simulink model "CFGOC_SSPUT02"  (R2023b)
settings: Solver=FixedStepAuto  StartTime=0.0  StopTime=400  RelTol=1e-3  EnableMultiTasking=on
undefined symbols (not defined in the file): Ta_p, Ta_x, Ta_y
libraries: mbedblockslib x11, simulink x10, mssSimulink x4, simulink_extras x2
settings Model: ExtModeTrigDuration=10  Creator=The MathWorks, Inc.  LastModifiedBy=Ly Soi
settings SolverCC: AlgebraicLoopSolver=TrustRegion  AutoInsertRateTranBlk=on  MaxZcPerStep=1
settings DataIOCC: ReturnWorkspaceOutputs=off
settings OptimizationCC: MaxStackSize=64
settings DebuggingCC: MultiTaskRateTransMsg=warning  ParameterTunabilityLossMsg=error  UnconnectedInputMsg=warning  UnconnectedOutputMsg=warning  UnconnectedLineMsg=warning  SubsystemReferenceDiagnosticForUnitTest=warning  ArithmeticOperatorsInVariantConditions=warning
settings HardwareCC: ProdBitPerPointer=32  ProdBitPerSizeT=32  ProdBitPerPtrDiffT=32  ProdLargestAtomicInteger=Long  ProdLargestAtomicFloat=Double  ProdWordSize=32  ProdLongLongMode=on  ProdHWDeviceType=ARM Compatible->ARM Cortex
settings ModelReferenceCC: EnableRefExpFcnMdlSchedulingChecks=on
settings SFSimCC: SimUseLocalCustomCode=off
settings RTWCC: Description=Embedded Coder  SystemTargetFile=ert.tlc  HardwareBoard=STM32 Nucleo F746ZG  TemplateMakefile=ert_default_tmf  GenerateReport=on  RTWUseLocalCustomCode=off  Toolchain=GNU Tools for ARM Embedded Processors  LaunchReport=on  DLArmComputeVersion=19.05
settings CodeAppCC: ForceParamTrailComments=on  OperatorAnnotations=on  StateflowObjectComments=on  MATLABSourceComments=on
settings ERTTargetCC: CodeReplacementLibrary=ARM Cortex-M (Optimized)  MultiwordLength=2048  ERTCustomFileBanners=off  SupportContinuousTime=on  SupportNonInlinedSFcns=on  RemoveResetFunc=off  ModelStepFunctionPrototypeControlCompliant=off  ExtModeTransport=3  ExtModeStaticAlloc=on  ExtModeStaticAllocSize=2000  ExtModeMexFile=ext_xcp  ExtModeIntrfLevel=Level2 - Open  ERTSrcFileBannerTemplate=codertarget_code_template.cgt  ERTHdrFileBannerTemplate=codertarget_code_template.cgt  ERTDataSrcFileTemplate=codertarget_code_template.cgt  ERTDataHdrFileTemplate=codertarget_code_template.cgt
settings ConfigComp: CovMetricSettings=dsw  CovSaveCumulativeToWorkspaceVar=on  CovSaveSingleToWorkspaceVar=on  CovExternalEMLEnable=off

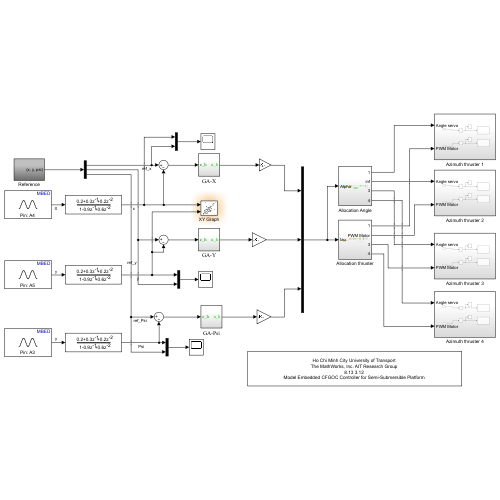
[thumbnail: Simulink's stored preview of the top-level diagram]
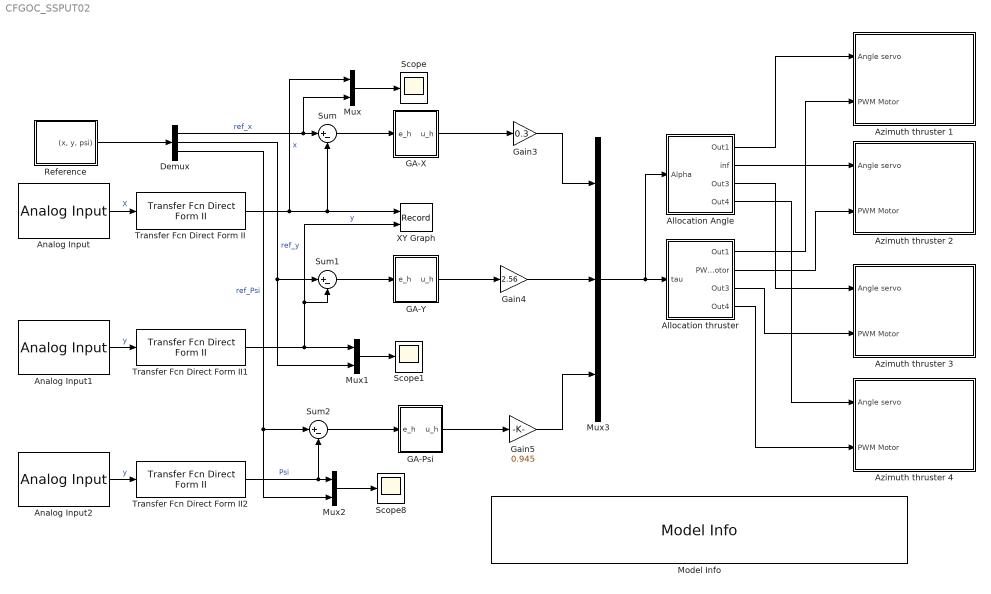
== system CFGOC_SSPUT02 ==
  Allocation Angle : Subsystem
  Allocation thruster : Subsystem
  Analog Input : mbedblockslib/Analog Input  Pin=A4  ReadResultsOnly=off  ConversionTriggerSource=Software  ExternalTriggerType=uint32( 0 )  OutputDataType=double  EnableConversionCompleteNotify=off  EnableOuputStatus=off  SampleTime=-1
      settings: LibrarySourceBlock=stmnucleorootlib/Common/Analog Input
  Analog Input1 : mbedblockslib/Analog Input  Pin=A5  ReadResultsOnly=off  ConversionTriggerSource=Software  ExternalTriggerType=uint32( 0 )  OutputDataType=double  EnableConversionCompleteNotify=off  EnableOuputStatus=off  SampleTime=-1
      settings: LibrarySourceBlock=stmnucleorootlib/Common/Analog Input
  Analog Input2 : mbedblockslib/Analog Input  Pin=A3  ReadResultsOnly=off  ConversionTriggerSource=Software  ExternalTriggerType=uint32( 0 )  OutputDataType=double  EnableConversionCompleteNotify=off  EnableOuputStatus=off  SampleTime=-1
      settings: LibrarySourceBlock=stmnucleorootlib/Common/Analog Input
  Azimuth thruster 1 : Subsystem
  Azimuth thruster 2 : Subsystem
  Azimuth thruster 3 : Subsystem
  Azimuth thruster 4 : Subsystem
  Demux : Demux  Outputs=3
  GA-Psi : Subsystem
  GA-X : Subsystem
  GA-Y : Subsystem
  Gain3 : Gain  Gain=0.3
  Gain4 : Gain  Gain=2.56
  Gain5 : Gain  Gain=0.945
  Model Info : simulink/Model-Wide Utilities/Model Info  Frame=on  DisplayStringWithTags=|  HorizontalTextAlignment=Center  LeftAlignmentValue=0.5
      | Ho Chi Minh City University of Transport
      | %<Creator> AIT Research Group
      | %<ModelVersion> 3.12
      | Model Embedded CFGOC Controller for Semi-Submersible Platform
  Mux : Mux  Inputs=2
  Mux1 : Mux  Inputs=2
  Mux2 : Mux  Inputs=2
  Mux3 : Mux  Inputs=3
  Reference : Subsystem
  Scope : Scope
  Scope1 : Scope
  Scope8 : Scope
  Sum : Sum  Inputs=|+-
  Sum1 : Sum  Inputs=|+-
  Sum2 : Sum  Inputs=|+-
  Transfer Fcn Direct Form II : simulink/Additional Math & Discrete/Additional Discrete/Transfer Fcn Direct Form II  NumCoefVec=[0.2 0.3 0.2]  DenCoefVec="[-0.9    0.6]"  vinit=0.0  DoSatur=off
  Transfer Fcn Direct Form II1 : simulink/Additional Math & Discrete/Additional Discrete/Transfer Fcn Direct Form II  NumCoefVec=[0.2 0.3 0.2]  DenCoefVec="[-0.9    0.6]"  vinit=0.0  DoSatur=off
  Transfer Fcn Direct Form II2 : simulink/Additional Math & Discrete/Additional Discrete/Transfer Fcn Direct Form II  NumCoefVec=[0.2 0.3 0.2]  DenCoefVec="[-0.9    0.6]"  vinit=0.0  DoSatur=off
  XY Graph : Record  FileSettingsInternal="{\"entries\":[{\"content\":{\"excelSettings\":{\"content\":{},\"type\":\"Streamout.ExcelSettings\"}},\"type\":\"Streamout.FileSettingStorage\",\"uuid\":\"\"}],\"packageUris\":[\"http:\\/\\/schema.mathworks.com\\/mf0\\/streamout_blocks\\/R2020a\"],\"version\":\"1.0\"}"  Layout=[1 1]  SignalsInternal="{\"entries\":[{\"content\":{\"signals\":[{\"content\":{\"blockPath\":[],\"dimensions\":[1],\"domain\":\"\",\"lineColor\":\"#a2142f\",\"plots\":[1],\"port\":1,\"signalID\":71,\"signalName\":\"Gain2\"},\"type\":\"RecordBlkView.Signal\",\"uuid\":\"\"},{\"content\":{\"blockPath\":[],\"dimensions\":[1],\"domain\":\"\",\"lineColor\":\"#139fff\",\"plots\":[1],\"port\":2,\"signalID\":74,\"signalName\":\"y\"},\"type\":\"RecordBlkView.Signal\",\"uuid\":\"\"}]},\"type\":\"RecordBlkView.InputSignals\",\"uuid\":\"\"}],\"packageUris\":[\"http:\\/\\/schema.mathworks.com\\/mf0\\/streamout_blocks\\/R2020a\"],\"version\":\"1.0\"}"  VisualizationBindings="{\"xyplotplugin\":{\"info\":[{\"series\":[{\"bindingParametersList\":[{\"parameter\":\"X-Axis\",\"signalID\":71,\"signalName\":\"Gain2\"},{\"parameter\":\"Y-Axis\",\"signalID\":74,\"signalName\":\"y\"}],\"seriesID\":16081}],\"subplotID\":1}]}}"  CompatibilityTag=XY
  wires:
  Analog Input/1 -> Transfer Fcn Direct Form II/1  "X"
  Analog Input1/1 -> Transfer Fcn Direct Form II1/1  "y"
  Demux/1 -> Mux/2, Sum/1  "ref_x"
  Demux/2 -> Mux1/2, Sum1/1  "ref_y"
  Mux/1 -> Scope/1
  Mux1/1 -> Scope1/1
  Transfer Fcn Direct Form II/1 -> Sum/2, XY Graph/1, Mux/1  "x"
  Transfer Fcn Direct Form II1/1 -> Mux1/1, XY Graph/2, Sum1/2  "y"
  GA-Psi/1(u_h) -> Gain5/1
  Sum/1 -> GA-X/1(e_h)
  Gain5/1 -> Mux3/3
  GA-Y/1(u_h) -> Gain4/1
  GA-X/1(u_h) -> Gain3/1
  Sum1/1 -> GA-Y/1(e_h)
  Gain3/1 -> Mux3/1
  Gain4/1 -> Mux3/2
  Transfer Fcn Direct Form II2/1 -> Sum2/2, Mux2/1  "Psi"
  Mux2/1 -> Scope8/1
  Analog Input2/1 -> Transfer Fcn Direct Form II2/1  "y"
  Demux/3 -> Sum2/1, Mux2/2  "ref_Psi"
  Sum2/1 -> GA-Psi/1(e_h)
  Mux3/1 -> Allocation Angle/1(Alpha), Allocation thruster/1(tau)
  Allocation Angle/1(Out1) -> Azimuth thruster 1/1(Angle servo)
  Allocation thruster/1(Out1) -> Azimuth thruster 1/2(PWM Motor)
  Allocation Angle/2(inf) -> Azimuth thruster 2/1(Angle servo)
  Allocation thruster/2(PWM Motor) -> Azimuth thruster 2/2(PWM Motor)
  Allocation Angle/3(Out3) -> Azimuth thruster 3/1(Angle servo)
  Allocation thruster/3(Out3) -> Azimuth thruster 3/2(PWM Motor)
  Allocation Angle/4(Out4) -> Azimuth thruster 4/1(Angle servo)
  Allocation thruster/4(Out4) -> Azimuth thruster 4/2(PWM Motor)
  Reference/1("(x, y, psi)") -> Demux/1

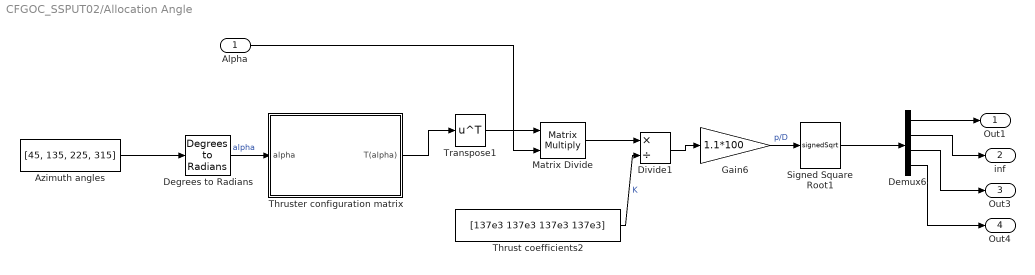
== system CFGOC_SSPUT02/Allocation Angle ==
  Alpha : Inport
  Azimuth angles : Constant  Value=[45, 135, 225, 315]
  Degrees to Radians : simulink_extras/Transformations/Degrees to Radians
  Demux6 : Demux
      settings: DisplayOption=none
  Divide1 : Product  Inputs=*/
  Gain6 : Gain  Gain=1.1*100  SaturateOnIntegerOverflow=on  OutDataTypeStr=Inherit: Same as input  ParamDataTypeStr=Inherit: Same as input
  Matrix Divide : Product  Inputs=**  Multiplication=Matrix(*)
  Signed Square Root1 : Sqrt  Operator=signedSqrt
  Thrust coefficients2 : Constant  Value=[137e3 137e3 137e3 137e3]
  "Thruster configuration matrix  " : Subsystem  AncestorBlock=mssSimulink/Modelling/Propulsion/Actuator Configuration/Thruster configuration matrix
  Transpose1 : Math  Operator=transpose
  Out1 : Outport
  inf : Outport  Port=2
  Out3 : Outport  Port=3
  Out4 : Outport  Port=4
  wires:
  Matrix Divide/1 -> Divide1/1
  Degrees to Radians/1 -> "Thruster configuration matrix  "/1(alpha)  "alpha"
  Signed Square Root1/1 -> Demux6/1
  Gain6/1 -> Signed Square Root1/1  "p/D"
  Azimuth angles/1 -> Degrees to Radians/1
  Thrust coefficients2/1 -> Divide1/2  "K"
  Transpose1/1 -> Matrix Divide/1
  Demux6/4 -> Out4/1
  Divide1/1 -> Gain6/1
  "Thruster configuration matrix  "/1(T(alpha)) -> Transpose1/1
  Alpha/1 -> Matrix Divide/2
  Demux6/1 -> Out1/1
  Demux6/3 -> Out3/1
  Demux6/2 -> inf/1

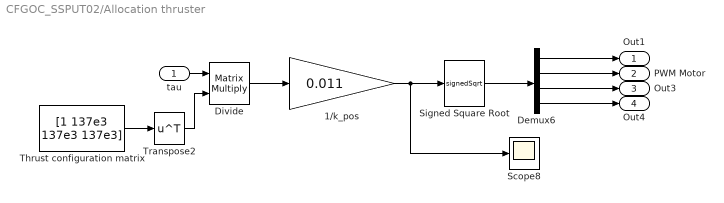
== system CFGOC_SSPUT02/Allocation thruster ==
  tau : Inport
  1/k_pos : Gain  Gain=0.011
  Demux6 : Demux
      settings: DisplayOption=none
  Divide : Product  Inputs=**  Multiplication=Matrix(*)
  Scope8 : Scope
  Signed Square Root : Sqrt  Operator=signedSqrt
  Thrust configuration matrix : Constant  Value=[1 137e3 137e3 137e3]
  Transpose2 : Math  Operator=transpose
  Out1 : Outport
  PWM Motor : Outport  Port=2
  Out3 : Outport  Port=3
  Out4 : Outport  Port=4
  wires:
  1/k_pos/1 -> Scope8/1, Signed Square Root/1
  Signed Square Root/1 -> Demux6/1
  Demux6/2 -> PWM Motor/1
  Demux6/1 -> Out1/1
  Demux6/3 -> Out3/1
  Demux6/4 -> Out4/1
  Transpose2/1 -> Divide/2
  Thrust configuration matrix/1 -> Transpose2/1
  Divide/1 -> 1/k_pos/1
  tau/1 -> Divide/1

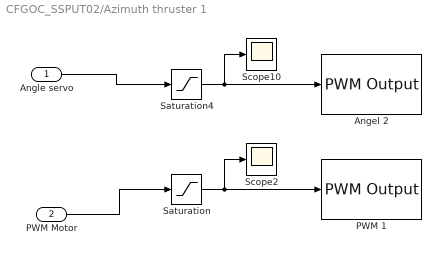
== system CFGOC_SSPUT02/Azimuth thruster 1 ==
  Angle servo : Inport
  PWM Motor : Inport  Port=2
  Angel 2 : mbedblockslib/PWM Output  Pin=D5  EnableInputFrequency=off  InitialFrequency=2000  InitialDutyCycle=50  NotificationType=None
      settings: LibrarySourceBlock=stmnucleorootlib/Common/PWM Output
  PWM 1 : mbedblockslib/PWM Output  Pin=D3  EnableInputFrequency=off  InitialFrequency=2000  InitialDutyCycle=50  NotificationType=None
      settings: LibrarySourceBlock=stmnucleorootlib/Common/PWM Output
  Saturation : Saturate  UpperLimit=255  LowerLimit=-255
  Saturation4 : Saturate  UpperLimit=255  LowerLimit=-255
  Scope10 : Scope
  Scope2 : Scope
  wires:
  Saturation/1 -> PWM 1/1, Scope2/1
  PWM Motor/1 -> Saturation/1
  Saturation4/1 -> Angel 2/1, Scope10/1
  Angle servo/1 -> Saturation4/1

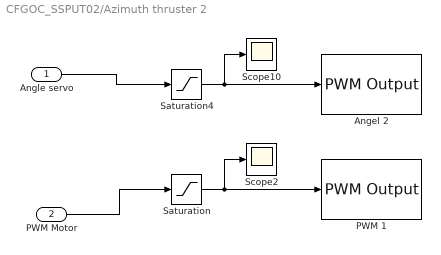
== system CFGOC_SSPUT02/Azimuth thruster 2 ==
  Angle servo : Inport
  PWM Motor : Inport  Port=2
  Angel 2 : mbedblockslib/PWM Output  Pin=D6  EnableInputFrequency=off  InitialFrequency=2000  InitialDutyCycle=50  NotificationType=None
      settings: LibrarySourceBlock=stmnucleorootlib/Common/PWM Output
  PWM 1 : mbedblockslib/PWM Output  Pin=D9  EnableInputFrequency=off  InitialFrequency=2000  InitialDutyCycle=50  NotificationType=None
      settings: LibrarySourceBlock=stmnucleorootlib/Common/PWM Output
  Saturation : Saturate  UpperLimit=255  LowerLimit=-255
  Saturation4 : Saturate  UpperLimit=255  LowerLimit=-255
  Scope10 : Scope
  Scope2 : Scope
  wires:
  Saturation/1 -> PWM 1/1, Scope2/1
  PWM Motor/1 -> Saturation/1
  Saturation4/1 -> Angel 2/1, Scope10/1
  Angle servo/1 -> Saturation4/1

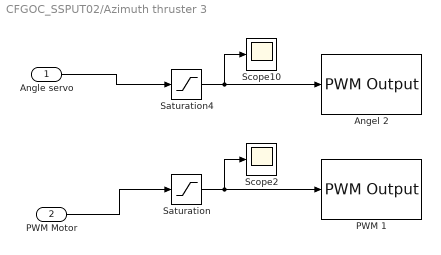
== system CFGOC_SSPUT02/Azimuth thruster 3 ==
  Angle servo : Inport
  PWM Motor : Inport  Port=2
  Angel 2 : mbedblockslib/PWM Output  Pin=D5  EnableInputFrequency=off  InitialFrequency=2000  InitialDutyCycle=50  NotificationType=None
      settings: LibrarySourceBlock=stmnucleorootlib/Common/PWM Output
  PWM 1 : mbedblockslib/PWM Output  Pin=D3  EnableInputFrequency=off  InitialFrequency=2000  InitialDutyCycle=50  NotificationType=None
      settings: LibrarySourceBlock=stmnucleorootlib/Common/PWM Output
  Saturation : Saturate  UpperLimit=255  LowerLimit=-255
  Saturation4 : Saturate  UpperLimit=255  LowerLimit=-255
  Scope10 : Scope
  Scope2 : Scope
  wires:
  Saturation/1 -> PWM 1/1, Scope2/1
  PWM Motor/1 -> Saturation/1
  Saturation4/1 -> Angel 2/1, Scope10/1
  Angle servo/1 -> Saturation4/1

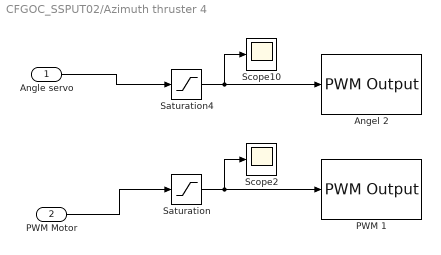
== system CFGOC_SSPUT02/Azimuth thruster 4 ==
  Angle servo : Inport
  PWM Motor : Inport  Port=2
  Angel 2 : mbedblockslib/PWM Output  Pin=D5  EnableInputFrequency=off  InitialFrequency=2000  InitialDutyCycle=50  NotificationType=None
      settings: LibrarySourceBlock=stmnucleorootlib/Common/PWM Output
  PWM 1 : mbedblockslib/PWM Output  Pin=D3  EnableInputFrequency=off  InitialFrequency=2000  InitialDutyCycle=50  NotificationType=None
      settings: LibrarySourceBlock=stmnucleorootlib/Common/PWM Output
  Saturation : Saturate  UpperLimit=255  LowerLimit=-255
  Saturation4 : Saturate  UpperLimit=255  LowerLimit=-255
  Scope10 : Scope
  Scope2 : Scope
  wires:
  Saturation/1 -> PWM 1/1, Scope2/1
  PWM Motor/1 -> Saturation/1
  Saturation4/1 -> Angel 2/1, Scope10/1
  Angle servo/1 -> Saturation4/1

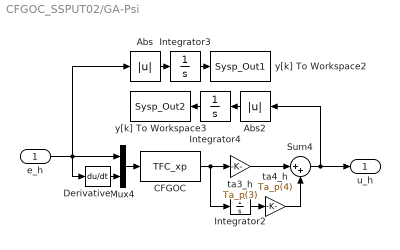
== system CFGOC_SSPUT02/GA-Psi ==
  e_h : Inport
  Abs : Abs  SaturateOnIntegerOverflow=off
  Abs2 : Abs  SaturateOnIntegerOverflow=off
  CFGOC : MATLABFcn  MATLABFcn=TFC_xp  OutputDimensions=1
  Derivative : Derivative
  Integrator2 : Integrator
  Integrator3 : Integrator
  Integrator4 : Integrator
  Mux4 : Mux  Inputs=2
  Sum4 : Sum  Inputs=|++  InputSameDT=on  SaturateOnIntegerOverflow=on  OutDataTypeStr=Inherit: Same as first input
  ta3_h : Gain  Gain=Ta_p(3)
  ta4_h : Gain  Gain=Ta_p(4)
  y[k] To Workspace2 : ToWorkspace  VariableName=Sysp_Out1  SaveFormat=Timeseries  SampleTime=-1
  y[k] To Workspace3 : ToWorkspace  VariableName=Sysp_Out2  SaveFormat=Timeseries  SampleTime=-1
  u_h : Outport
  wires:
  Sum4/1 -> u_h/1, Abs2/1
  Derivative/1 -> Mux4/2
  Mux4/1 -> CFGOC/1
  CFGOC/1 -> ta3_h/1, Integrator2/1
  Integrator2/1 -> ta4_h/1
  ta4_h/1 -> Sum4/2
  ta3_h/1 -> Sum4/1
  e_h/1 -> Abs/1, Derivative/1, Mux4/1
  Integrator3/1 -> y[k] To Workspace2/1
  Integrator4/1 -> y[k] To Workspace3/1
  Abs/1 -> Integrator3/1
  Abs2/1 -> Integrator4/1

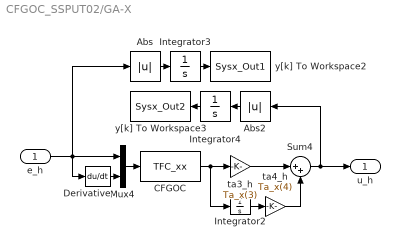
== system CFGOC_SSPUT02/GA-X ==
  e_h : Inport
  Abs : Abs  SaturateOnIntegerOverflow=off
  Abs2 : Abs  SaturateOnIntegerOverflow=off
  CFGOC : MATLABFcn  MATLABFcn=TFC_xx  OutputDimensions=1
  Derivative : Derivative
  Integrator2 : Integrator
  Integrator3 : Integrator
  Integrator4 : Integrator
  Mux4 : Mux  Inputs=2
  Sum4 : Sum  Inputs=|++  InputSameDT=on  SaturateOnIntegerOverflow=on  OutDataTypeStr=Inherit: Same as first input
  ta3_h : Gain  Gain=Ta_x(3)
  ta4_h : Gain  Gain=Ta_x(4)
  y[k] To Workspace2 : ToWorkspace  VariableName=Sysx_Out1  SaveFormat=Timeseries  SampleTime=-1
  y[k] To Workspace3 : ToWorkspace  VariableName=Sysx_Out2  SaveFormat=Timeseries  SampleTime=-1
  u_h : Outport
  wires:
  Sum4/1 -> u_h/1, Abs2/1
  Derivative/1 -> Mux4/2
  Mux4/1 -> CFGOC/1
  CFGOC/1 -> ta3_h/1, Integrator2/1
  Integrator2/1 -> ta4_h/1
  ta4_h/1 -> Sum4/2
  ta3_h/1 -> Sum4/1
  e_h/1 -> Abs/1, Derivative/1, Mux4/1
  Integrator3/1 -> y[k] To Workspace2/1
  Integrator4/1 -> y[k] To Workspace3/1
  Abs/1 -> Integrator3/1
  Abs2/1 -> Integrator4/1

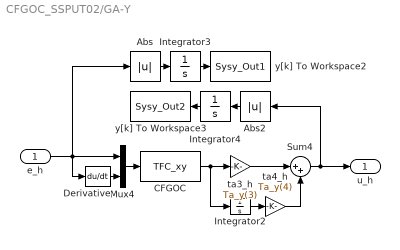
== system CFGOC_SSPUT02/GA-Y ==
  e_h : Inport
  Abs : Abs  SaturateOnIntegerOverflow=off
  Abs2 : Abs  SaturateOnIntegerOverflow=off
  CFGOC : MATLABFcn  MATLABFcn=TFC_xy  OutputDimensions=1
  Derivative : Derivative
  Integrator2 : Integrator
  Integrator3 : Integrator
  Integrator4 : Integrator
  Mux4 : Mux  Inputs=2
  Sum4 : Sum  Inputs=|++  InputSameDT=on  SaturateOnIntegerOverflow=on  OutDataTypeStr=Inherit: Same as first input
  ta3_h : Gain  Gain=Ta_y(3)
  ta4_h : Gain  Gain=Ta_y(4)
  y[k] To Workspace2 : ToWorkspace  VariableName=Sysy_Out1  SaveFormat=Timeseries  SampleTime=-1
  y[k] To Workspace3 : ToWorkspace  VariableName=Sysy_Out2  SaveFormat=Timeseries  SampleTime=-1
  u_h : Outport
  wires:
  Sum4/1 -> u_h/1, Abs2/1
  Derivative/1 -> Mux4/2
  Mux4/1 -> CFGOC/1
  CFGOC/1 -> ta3_h/1, Integrator2/1
  Integrator2/1 -> ta4_h/1
  ta4_h/1 -> Sum4/2
  ta3_h/1 -> Sum4/1
  e_h/1 -> Abs/1, Derivative/1, Mux4/1
  Integrator3/1 -> y[k] To Workspace2/1
  Integrator4/1 -> y[k] To Workspace3/1
  Abs/1 -> Integrator3/1
  Abs2/1 -> Integrator4/1

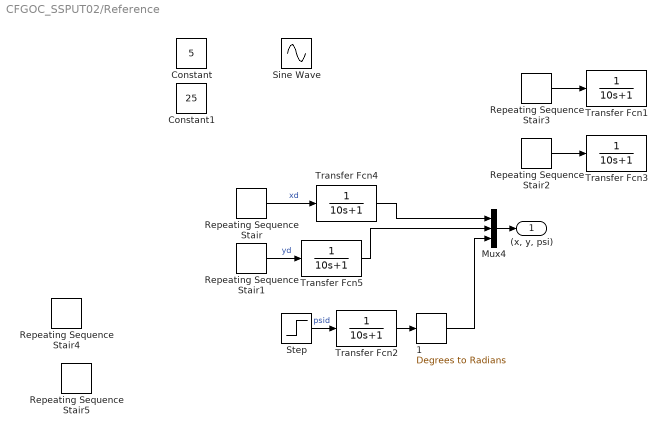
== system CFGOC_SSPUT02/Reference ==
  "     1" : simulink_extras/Transformations/Degrees to Radians
  Constant : Constant  Value=5
  Constant1 : Constant  Value=25
  Mux4 : Mux  Inputs=3
  Repeating Sequence Stair : simulink/Sources/Repeating Sequence Stair  OutValues=[10 0 10]  tsamp=100  OutMin=[]  OutMax=[]  OutDataTypeStr=double  OutputDataTypeScalingMode=double  OutDataType=fixdt(0,8)  ConRadixGroup=Best Precision: Vector-wise  OutScaling=2^-12
  Repeating Sequence Stair1 : simulink/Sources/Repeating Sequence Stair  OutValues=[0 10 10]  tsamp=100  OutMin=[]  OutMax=[]  OutDataTypeStr=double  OutputDataTypeScalingMode=double  OutDataType=fixdt(0,8)  ConRadixGroup=Best Precision: Vector-wise  OutScaling=2^-12
  Repeating Sequence Stair2 : simulink/Sources/Repeating Sequence Stair  OutValues=[7 -7 0 7]  tsamp=10  OutMin=[]  OutMax=[]  OutDataTypeStr=double  OutputDataTypeScalingMode=double  OutDataType=fixdt(0,8)  ConRadixGroup=Best Precision: Vector-wise  OutScaling=2^-12
  Repeating Sequence Stair3 : simulink/Sources/Repeating Sequence Stair  OutValues=[-7 7 0 7]  tsamp=10  OutMin=[]  OutMax=[]  OutDataTypeStr=double  OutputDataTypeScalingMode=double  OutDataType=fixdt(0,8)  ConRadixGroup=Best Precision: Vector-wise  OutScaling=2^-12
  Repeating Sequence Stair4 : simulink/Sources/Repeating Sequence Stair  OutValues="[0\t0\t0\t0\t0\t0\t0\t0\t0\t0\t0\t0\t0\t0\t0\t0\t0\t0\t0\t0\t0\t0\t0\t0\t0\t0\t0\t0\t0\t0\t0\t0\t0\t0\t0\t0\t0\t0\t0\t0\t0\t0\t0\t0\t0\t0\t0\t0\t0\t0\t0\t0\t0\t0\t0\t0\t0\t0\t0\t0\t0\t0\t0\t0\t0\t0\t0\t0\t0\t0\t0\t0\t0\t0\t0\t0\t0\t0\t0\t0\t0\t0\t0\t0\t0\t0\t0\t0\t0\t0\t0\t0\t0\t0\t0\t0\t0\t0\t0\t0\t0\t0\t0\t0.2\t0.4\t0.6\t0.8\t1\t1.2\t1.4\t1.6\t1.8\t2\t2.2\t2.4\t2.6\t2.8\t3\t3.2\t3.4\t3.6\t3.8\t4\t4.2\t4.4\t4.6\t4.8\t5\t5.2\t5.4\t5.6\t5.8\t6\t6.2\t6.4\t6.6\t6.8\t7\t7.2\t7.4\t7.6\t7.8\t8\t8.2\t8.4\t8.6\t8.8\t9\t9.2\t9.4\t9.6\t9.8\t10\t10\t10\t10\t10\t10\t10\t10\t10\t10\t10\t10\t10\t10\t10\t10\t10\t10\t10\t10\t10\t10\t10\t10\t10\t10\t10\t10\t10\t10\t10\t10\t10\t10\t10\t10\t10\t10\t10\t10\t10\t10\t10\t10\t10\t10\t10\t10\t10\t10\t10\t10]"  tsamp=1  OutMin=[]  OutMax=[]  OutDataTypeStr=double  OutputDataTypeScalingMode=double  OutDataType=fixdt(0,8)  ConRadixGroup=Best Precision: Vector-wise  OutScaling=2^-12
  Repeating Sequence Stair5 : simulink/Sources/Repeating Sequence Stair  OutValues="[0\t0.2\t0.4\t0.6\t0.8\t1\t1.2\t1.4\t1.6\t1.8\t2\t2.2\t2.4\t2.6\t2.8\t3\t3.2\t3.4\t3.6\t3.8\t4\t4.2\t4.4\t4.6\t4.8\t5\t5.2\t5.4\t5.6\t5.8\t6\t6.2\t6.4\t6.6\t6.8\t7\t7.2\t7.4\t7.6\t7.8\t8\t8.2\t8.4\t8.6\t8.8\t9\t9.2\t9.4\t9.6\t9.8\t10\t10\t10\t10\t10\t10\t10\t10\t10\t10\t10\t10\t10\t10\t10\t10\t10\t10\t10\t10\t10\t10\t10\t10\t10\t10\t10\t10\t10\t10\t10\t10\t10\t10\t10\t10\t10\t10\t10\t10\t10\t10\t10\t10\t10\t10\t10\t10\t10\t10\t10\t10\t10\t10\t10\t10\t10\t10\t10\t10\t10\t10\t10\t10\t10\t10\t10\t10\t10\t10\t10\t10\t10\t10\t10\t10\t10\t10\t10\t10\t10\t10\t10\t10\t10\t10\t10\t10\t10\t10\t10\t10\t10\t10\t10\t10\t10\t10\t10\t10\t10\t10\t10\t10\t10\t10\t10\t10\t10\t10\t10\t10\t10\t10\t10\t10\t10\t10\t10\t10\t10\t10\t10\t10\t10\t10\t10\t10\t10\t10\t10\t10\t10\t10\t10\t10\t10\t10\t10\t10\t10\t10\t10\t10\t10\t10\t10\t10\t10\t10\t10\t10\t10\t10]"  tsamp=1  OutMin=[]  OutMax=[]  OutDataTypeStr=double  OutputDataTypeScalingMode=double  OutDataType=fixdt(0,8)  ConRadixGroup=Best Precision: Vector-wise  OutScaling=2^-12
  Sine Wave : Sin  Frequency=4  SampleTime=0
  Step : Step  Time=0  After=20  SampleTime=0
  Transfer Fcn{1..5} (5 alike) : TransferFcn  Denominator=[10 1]
  "(x, y, psi)" : Outport
  wires:
  Mux4/1 -> "(x, y, psi)"/1
  "     1"/1 -> Mux4/3
  Step/1 -> Transfer Fcn2/1  "psid"
  Transfer Fcn2/1 -> "     1"/1
  Repeating Sequence Stair2/1 -> Transfer Fcn3/1
  Repeating Sequence Stair3/1 -> Transfer Fcn1/1
  Repeating Sequence Stair/1 -> Transfer Fcn4/1  "xd"
  Repeating Sequence Stair1/1 -> Transfer Fcn5/1  "yd"
  Transfer Fcn4/1 -> Mux4/1
  Transfer Fcn5/1 -> Mux4/2

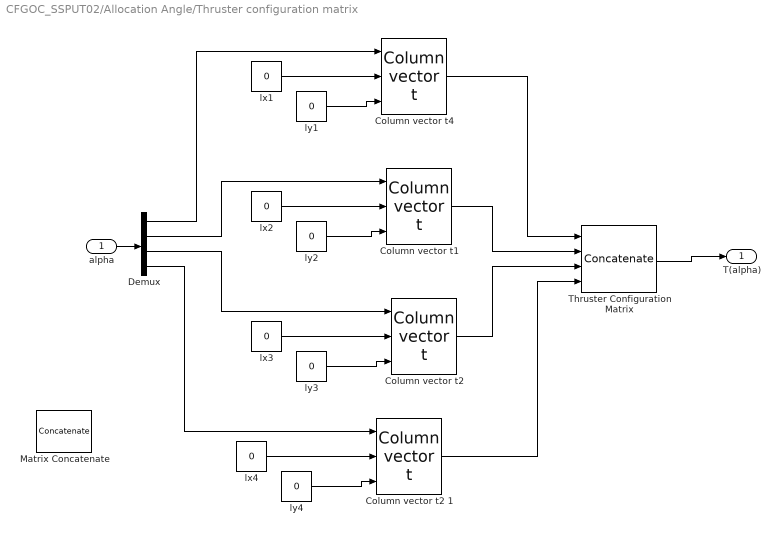
== system CFGOC_SSPUT02/Allocation Angle/Thruster configuration matrix   ==
  alpha : Inport
  "Column vector t1 " : mssSimulink/Modelling/Propulsion/Actuator Configuration/Column vector t  SystemSampleTime=-1  VariantActivationTime=update diagram  AllowFlexibleInterface=on  Latency=0  AutoFrameSizeCalculation=off
  "Column vector t2 " : mssSimulink/Modelling/Propulsion/Actuator Configuration/Column vector t  SystemSampleTime=-1  VariantActivationTime=update diagram  AllowFlexibleInterface=on  Latency=0  AutoFrameSizeCalculation=off
  Column vector t2 1 : mssSimulink/Modelling/Propulsion/Actuator Configuration/Column vector t  SystemSampleTime=-1  VariantActivationTime=update diagram  AllowFlexibleInterface=on  Latency=0  AutoFrameSizeCalculation=off
  "Column vector t4 " : mssSimulink/Modelling/Propulsion/Actuator Configuration/Column vector t  SystemSampleTime=-1  VariantActivationTime=update diagram  AllowFlexibleInterface=on  Latency=0  AutoFrameSizeCalculation=off
  Demux : Demux
      settings: DisplayOption=none
  Matrix Concatenate : Concatenate  NumInputs=1  Mode=Multidimensional array  ConcatenateDimension=4
  Thruster Configuration Matrix : Concatenate  NumInputs=4  Mode=Multidimensional array  ConcatenateDimension=2
  lx{1..4} (4 alike) : Constant  Value=0
  ly{1..4} (4 alike) : Constant  Value=0
  T(alpha) : Outport  VectorParamsAs1DForOutWhenUnconnected=off
  wires:
  ly3/1 -> "Column vector t2 "/3
  lx3/1 -> "Column vector t2 "/2
  ly2/1 -> "Column vector t1 "/3
  lx2/1 -> "Column vector t1 "/2
  ly1/1 -> "Column vector t4 "/3
  lx1/1 -> "Column vector t4 "/2
  Thruster Configuration Matrix/1 -> T(alpha)/1
  alpha/1 -> Demux/1
  Demux/3 -> "Column vector t2 "/1
  Demux/2 -> "Column vector t1 "/1
  Demux/1 -> "Column vector t4 "/1
  "Column vector t2 "/1 -> Thruster Configuration Matrix/3
  "Column vector t1 "/1 -> Thruster Configuration Matrix/2
  "Column vector t4 "/1 -> Thruster Configuration Matrix/1
  ly4/1 -> Column vector t2 1/3
  lx4/1 -> Column vector t2 1/2
  Demux/4 -> Column vector t2 1/1
  Column vector t2 1/1 -> Thruster Configuration Matrix/4
